simulink model "superhet_hw"  (R2021b)
settings: Solver=VariableStepAuto  StartTime=0.0  StopTime=0.1  RelTol=1e-3
libraries: dsparch4 x2
settings Model: Creator=EternoPax  LastModifiedBy=EternoPax

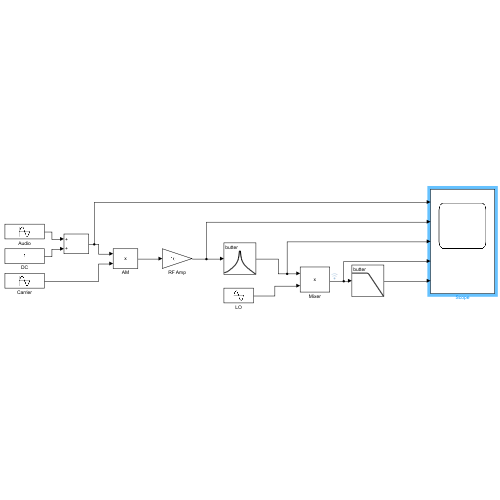
[thumbnail: Simulink's stored preview of the top-level diagram]
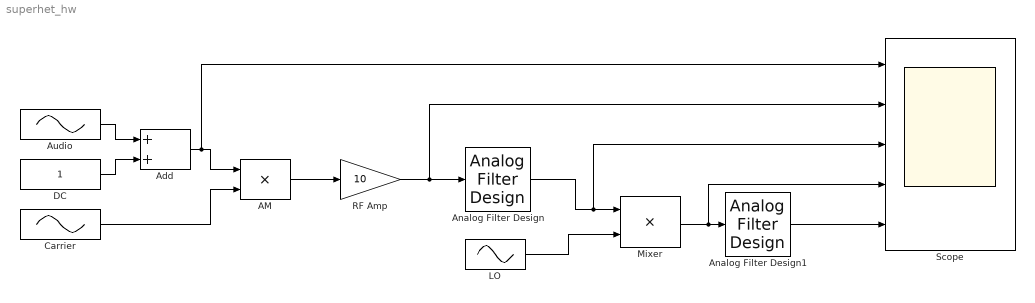
== system superhet_hw ==
  AM : Product
  Add : Sum
  Analog Filter Design : dsparch4/Analog Filter Design  method=Butterworth  filttype=Bandpass  N=8  Wlo=998000  Whi=1002000  Rp=2  Rs=40
  Analog Filter Design1 : dsparch4/Analog Filter Design  method=Butterworth  filttype=Lowpass  N=8  Wlo=2000  Whi=1002000  Rp=2  Rs=40
  Audio : Sin  Amplitude=0.8  Frequency=1000  SampleTime=0
  Carrier : Sin  Frequency=1000000  SampleTime=0
  DC : Constant
  LO : Sin  Frequency=1000000  SampleTime=0
  Mixer : Product
  RF Amp : Gain  Gain=10
  Scope : Scope  NumInputPorts=5
  wires:
  Audio/1 -> Add/1
  DC/1 -> Add/2
  Add/1 -> Scope/1, AM/1
  Carrier/1 -> AM/2
  AM/1 -> RF Amp/1
  LO/1 -> Mixer/2
  RF Amp/1 -> Scope/2, Analog Filter Design/1
  Analog Filter Design/1 -> Scope/3, Mixer/1
  Mixer/1 -> Scope/4, Analog Filter Design1/1
  Analog Filter Design1/1 -> Scope/5
